simulink library "SOMANET"  (R2016b)
settings: Solver=VariableStepAuto  StartTime=0.0  StopTime=10.0  RelTol=1e-3
undefined symbols (not defined in the file): SomanetError
libraries: simulink x1, ConfigHandler x1, SafetyCheckerSOMANET x1, SubsystemEnabler x1, TuningHandler x1, StatemachineSOMANET x1
settings Model: Creator=Nathan  LastModifiedBy=march

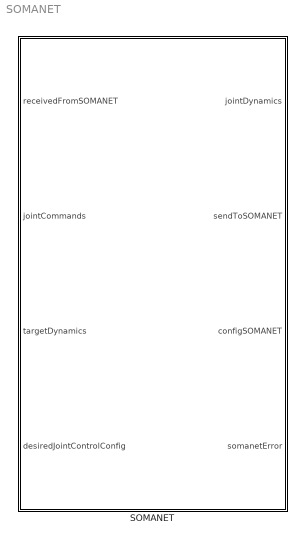
== system SOMANET ==
  SOMANET : Subsystem

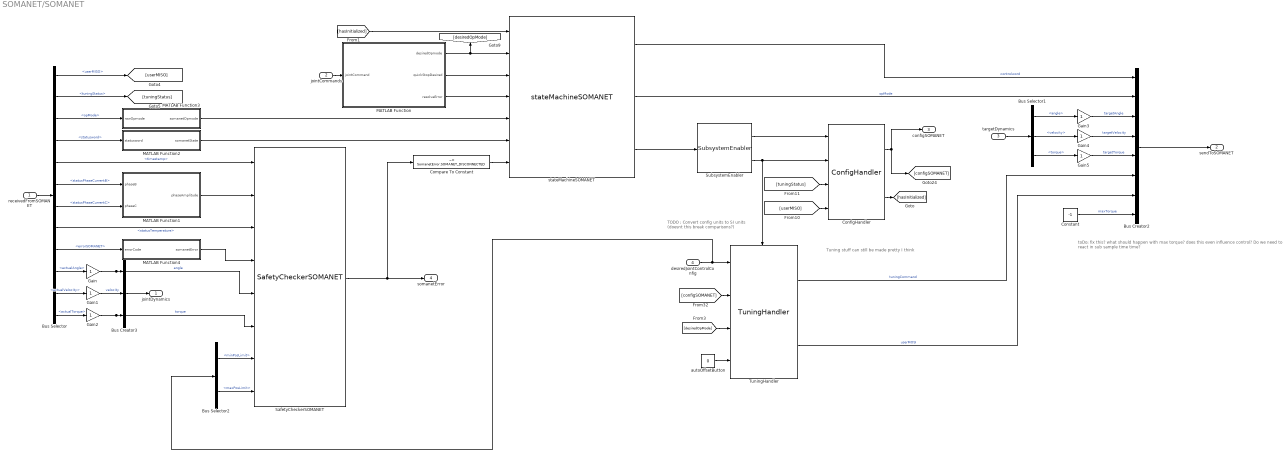
== system SOMANET/SOMANET ==
  note: TODO : Convert config units to SI units
      | (doesnt this break comparisons?)
  note: toDo: fix this? what should happen with max torque? does this even influence control? Do we need to react in sub sample time time?
  note: Tuning stuff can still be made pretty I think
  receivedFromSOMANET : Inport  OutDataTypeStr=Bus: EtherCATReceivedFromSOMANET  BusOutputAsStruct=on
  jointCommands : Inport  Port=2
  targetDynamics : Inport  Port=3  OutDataTypeStr=Bus: JointDynamics  BusOutputAsStruct=on
  desiredJointControlConfig : Inport  Port=4  OutDataTypeStr=Bus: JointControlConfig
  Bus Creator2 : BusCreator  Inputs=8  OutDataTypeStr=Bus: EtherCATSendToSOMANET  NonVirtualBus=on
  Bus Creator3 : BusCreator  Inputs=3  OutDataTypeStr=Bus: JointDynamics  NonVirtualBus=on
  Bus Selector : BusSelector  OutputSignals=userMISO,tuningStatus,opMode,statusword,timestamp,statusPhaseCurrentB,statusPhaseCurrentC,statusTemperature,errorSOMANET,actualAngle,actualVelocity,actualTorque
  Bus Selector1 : BusSelector  OutputSignals=angle,velocity,torque
  Bus Selector2 : BusSelector  OutputSignals=minPosLimit,maxPosLimit
  Compare To Constant : simulink/Logic and Bit Operations/Compare To Constant  relop=~=  const=SomanetError.SOMANET_DISCONNECTED  OutDataTypeStr=boolean
  ConfigHandler : ConfigHandler/ConfigHandler
  Constant : Constant  Value=-1
  Gain{,1..5} (6 alike) : Gain
  MATLAB Function : MATLAB Function  TreatAsAtomicUnit=on
  MATLAB Function1 : MATLAB Function  TreatAsAtomicUnit=on
  MATLAB Function2 : MATLAB Function  TreatAsAtomicUnit=on
  MATLAB Function3 : MATLAB Function  TreatAsAtomicUnit=on
  MATLAB Function4 : MATLAB Function  TreatAsAtomicUnit=on
  SafetyCheckerSOMANET : SafetyCheckerSOMANET/SafetyCheckerSOMANET
  SubsystemEnabler : SubsystemEnabler/SubsystemEnabler
  TuningHandler : TuningHandler/TuningHandler
  autoOffsetButton : Constant  Value=0
  stateMachineSOMANET : StatemachineSOMANET/stateMachineSOMANET
  jointDynamics : Outport  OutDataTypeStr=Bus: JointDynamics
  sendToSOMANET : Outport  Port=2  OutDataTypeStr=Bus: EtherCATSendToSOMANET  BusOutputAsStruct=on
  configSOMANET : Outport  Port=3  OutDataTypeStr=Bus: JointControlConfig  BusOutputAsStruct=on
  somanetError : Outport  Port=4  OutDataTypeStr=Enum: SomanetError
  wires:
  Gain5/1 -> Bus Creator2/5  "targetTorque"
  Gain3/1 -> Bus Creator2/3  "targetAngle"
  Gain4/1 -> Bus Creator2/4  "targetVelocity"
  Bus Selector1/3 -> Gain5/1  "<torque>"
  Bus Selector1/1 -> Gain3/1  "<angle>"
  Bus Selector1/2 -> Gain4/1  "<velocity>"
  Gain2/1 -> Bus Creator3/3, SafetyCheckerSOMANET/6  "torque"
  Gain1/1 -> Bus Creator3/2  "velocity"
  Gain/1 -> Bus Creator3/1, SafetyCheckerSOMANET/5  "angle"
  Bus Selector/9 -> MATLAB Function4/1(errorCode)  "<errorSOMANET>"
  Bus Selector/8 -> SafetyCheckerSOMANET/3  "<statusTemperature>"
  Bus Selector/6 -> MATLAB Function1/1(phaseB)  "<statusPhaseCurrentB>"
  Bus Selector/7 -> MATLAB Function1/2(phaseC)  "<statusPhaseCurrentC>"
  Bus Selector/5 -> SafetyCheckerSOMANET/1  "<timestamp>"
  Bus Selector/4 -> MATLAB Function2/1(statusword)  "<statusword>"
  Bus Selector/3 -> MATLAB Function3/1(rawOpmode)  "<opMode>"
  [hasInitialized] -> stateMachineSOMANET/1
  SafetyCheckerSOMANET/1 -> somanetError/1, Compare To Constant/1
  jointCommands/1 -> MATLAB Function/1(jointCommand)
  autoOffsetButton/1 -> TuningHandler/4
  [configSOMANET] -> TuningHandler/2
  [desiredOpMode] -> TuningHandler/3
  stateMachineSOMANET/3 -> SubsystemEnabler/1
  SubsystemEnabler/2 -> ConfigHandler/2, TuningHandler/Enable
  SubsystemEnabler/1 -> ConfigHandler/1
  ConfigHandler/2 -> [hasInitialized]
  [tuningStatus] -> ConfigHandler/3
  [userMISO] -> ConfigHandler/4
  ConfigHandler/1 -> configSOMANET/1, [configSOMANET]
  Bus Creator2/1 -> sendToSOMANET/1
  Bus Selector/1 -> [userMISO]  "<userMISO>"
  stateMachineSOMANET/2 -> Bus Creator2/2  "opMode"
  TuningHandler/2 -> Bus Creator2/7  "userMOSI"
  TuningHandler/1 -> Bus Creator2/6  "tuningCommand"
  stateMachineSOMANET/1 -> Bus Creator2/1  "controlword"
  receivedFromSOMANET/1 -> Bus Selector/1
  Bus Selector/2 -> [tuningStatus]  "<tuningStatus>"
  Constant/1 -> Bus Creator2/8  "maxTorque"
  MATLAB Function3/1(somanetOpmode) -> stateMachineSOMANET/5
  MATLAB Function/3(resolveError) -> stateMachineSOMANET/4
  MATLAB Function2/1(somanetState) -> stateMachineSOMANET/6
  MATLAB Function/1(desiredOpmode) -> [desiredOpMode], stateMachineSOMANET/2
  Compare To Constant/1 -> stateMachineSOMANET/7
  MATLAB Function/2(quickStopDesired) -> stateMachineSOMANET/3
  Bus Creator3/1 -> jointDynamics/1
  Bus Selector/12 -> Gain2/1  "<actualTorque>"
  Bus Selector/11 -> Gain1/1  "<actualVelocity>"
  Bus Selector/10 -> Gain/1  "<actualAngle>"
  desiredJointControlConfig/1 -> TuningHandler/1, Bus Selector2/1
  Bus Selector2/1 -> SafetyCheckerSOMANET/7  "<minPosLimit>"
  Bus Selector2/2 -> SafetyCheckerSOMANET/8  "<maxPosLimit>"
  targetDynamics/1 -> Bus Selector1/1
  MATLAB Function1/1(phaseAmplitude) -> SafetyCheckerSOMANET/2
  MATLAB Function4/1(somanetError) -> SafetyCheckerSOMANET/4

== matlab function SOMANET/MATLAB Function ==
  data: jointCommand input; desiredOpmode output; quickStopDesired output; resolveError output
function [desiredOpmode, quickStopDesired, resolveError] = getSomanetCommands(jointCommand)
% jointCommand should be some enum
% with possible values something like:
%   * torqueControl
%   * positionControl
%   * velocityControl
%   * deactivateMotors
%   * resetError (?)
%   * don't move
% from these commands, the desired control words/opmodes/quick stops/
% whatever can be derived.
% point of this is that the master can be agnostic about the precise
% control mechanism of the somanet
persistent prevOpmode;
if(isempty(prevOpmode))
    prevOpmode = SomanetOpmode.CSTORQUE;
end

switch jointCommand
    case JointCommand.POSITIONCONTROL
        desiredOpmode = SomanetOpmode.CSPOSITION;
        quickStopDesired = 0;
        resolveError = 0;
    case JointCommand.VELOCITYCONTROL
        desiredOpmode = SomanetOpmode.CSVELOCITY;
        quickStopDesired = 0;
        resolveError = 0;
    case JointCommand.TORQUECONTROL
        desiredOpmode = SomanetOpmode.CSTORQUE;
        quickStopDesired = 0;
        resolveError = 0;
    case JointCommand.RESOLVEERROR
        desiredOpmode = prevOpmode;
        quickStopDesired = 0;
        resolveError = 1;
    otherwise
        desiredOpmode = SomanetOpmode.CSTORQUE;
        quickStopDesired = 1;
        resolveError = 0;
end

% update persistent variables
prevOpmode = desiredOpmode;
end

== matlab function SOMANET/MATLAB Function1 ==
  data: phaseB input; phaseAmplitude output; phaseC input
function phaseAmplitude = getPhaseAmplitude( phaseB, phaseC )
% wrapper function for getPhaseAmplitude
[ phaseAmplitude ] = getPhaseAmplitude( phaseB, phaseC );
end

== matlab function SOMANET/MATLAB Function2 ==
  data: statusword input; somanetState output
function somanetState = getSomanetState( statusword )
% wrapper function for getSomanetState
somanetState = getSomanetState( statusword );
end

== matlab function SOMANET/MATLAB Function3 ==
  data: rawOpmode input; somanetOpmode output
function somanetOpmode   = getSomanetOpmode( rawOpmode )
% wrapper function for getSomanetOpmode
somanetOpmode = getSomanetOpmode(rawOpmode);
end

== matlab function SOMANET/MATLAB Function4 ==
  data: errorCode input; somanetError output
function somanetError  = getErrorFromErrorCode(errorCode)
% wrapper for getErrorFromErroCode
somanetError = getErrorFromErrorCode(errorCode);
end
